simulink model "simulinkw2"  (R2024a)
settings: Solver=VariableStepAuto  StartTime=0.0  StopTime=10.0  RelTol=1e-3
values from neighbouring files (symbols this model uses):
  polyden = poly([-2 ; -3 ; -4 ])    [Week2.m]
  Polynum = 1    [Week2.m]
settings Model: Creator=mohammed  LastModifiedBy=mohammed

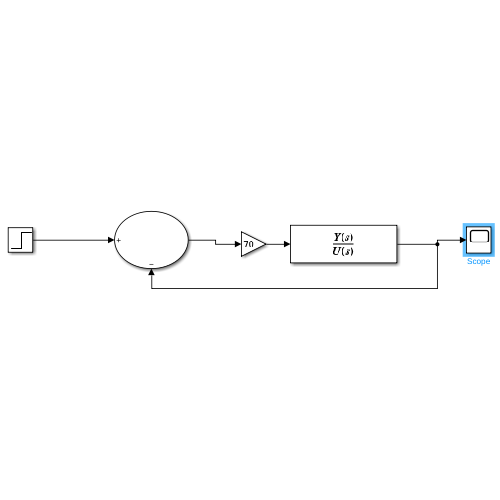
[thumbnail: Simulink's stored preview of the top-level diagram]
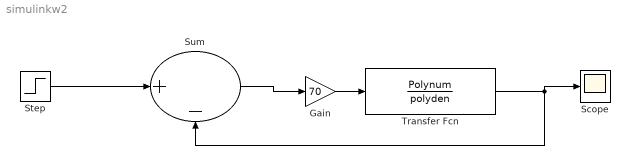
== system simulinkw2 ==
  Gain : Gain  Gain=70
  Scope : Scope
  Step : Step  Time=0  SampleTime=0
  Sum : Sum  Inputs=|+-
  Transfer Fcn : TransferFcn  Numerator=Polynum  Denominator=polyden
  wires:
  Step/1 -> Sum/1
  Transfer Fcn/1 -> Scope/1, Sum/2
  Gain/1 -> Transfer Fcn/1
  Sum/1 -> Gain/1
